simulink model "cordic_test"  (Simulink 6.1)
settings: Solver=FixedStepDiscrete  StartTime=0.0  StopTime=22000.0  FixedStep=1  RelTol=1e-3
libraries: simulink x1, modelsimlib x1
settings Model: LastModifiedBy=user
settings DebuggingCC: SolverPrmCheckMsg=warning

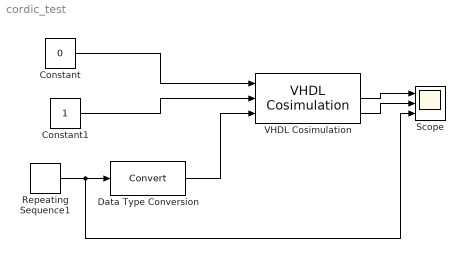
== system cordic_test ==
  Constant : Constant  Value=0  OutDataTypeMode=boolean  SampleTime=1
  Constant1 : Constant  OutDataTypeMode=boolean  SampleTime=1
  Data Type Conversion : DataTypeConversion  OutDataTypeMode=Specify via dialog  OutDataType=sfrac(16,2)  RndMeth=Nearest  SampleTime=1  SaturateOnIntegerOverflow=on
  Repeating Sequence1 : simulink/Sources/Repeating Sequence  rep_seq_t=[0 20000]  rep_seq_y=[-pi pi]
  Scope : Scope  NumInputPorts=3
      settings: TimeRange=25000  YMin=-5~-1~-5  YMax=5~1~5  MaxDataPoints=120000
  VHDL Cosimulation : modelsimlib/VHDL Cosimulation  DialogController=modelsimddg.CoSim  DialogControllerArgs=DataTag0  PortPaths=/cordic/rst;/cordic/run;/cordic/angle;/cordic/done;/cordic/sin;/cordic/cos  PortModes=[1 1 1 2 2 2 ]  PortTimes=[-1 -1 -1 -1 -1 -1 ]  PortSigns=[-1 -1 -1 -1 1 1 ]  PortFracLengths=[0 0 0 0 13 13 ]  CommLocal=on  CommSharedMemory=on  CommPortNumber=4449  CommShowInfo=on  ClockPaths=/cordic/clk  ClockModes=[2 ]  ClockTimes=[10 ]  TclPreSimCommand="echo \"Running Simulink Cosimulation block.\""  idxCellArray={'UNUSED_VAR'}
  wires:
  Constant/1 -> VHDL Cosimulation/1
  Constant1/1 -> VHDL Cosimulation/2
  Data Type Conversion/1 -> VHDL Cosimulation/3
  Repeating Sequence1/1 -> Data Type Conversion/1, Scope/3
  VHDL Cosimulation/2 -> Scope/1
  VHDL Cosimulation/3 -> Scope/2
